simulink model "quaternion_attitude_control_nominal"  (R2024b)
settings: Solver=ode45  StartTime=0.0  StopTime=1500  MaxStep=0.2
values from neighbouring files (symbols this model uses):
  Cross_section_area = 0.01    [init_conditions.m]
  d = 0.8    [init_conditions.m]
  finalAttitude = [-1/sqrt(2); 0; 0; -1/sqrt(2)]    [init_conditions.m]
  J = calculateInertiaTensor(mass, sideLength)    [init_conditions.m]
  k = 0.32    [init_conditions.m]
  mass = 1.33    [init_conditions.m]
undefined symbols (not defined in the file or in its folder): compute_drag
libraries: aerolibutil x2, aerolibgravity2 x1
settings Model: VariantFading=off  LastModifiedBy=shavykashyap
settings SolverCC: ZeroCrossAlgorithm=Adaptive
settings DataIOCC: Refine=2
settings DebuggingCC: MaskedZcDiagnostic=none  IgnoredZcDiagnostic=none

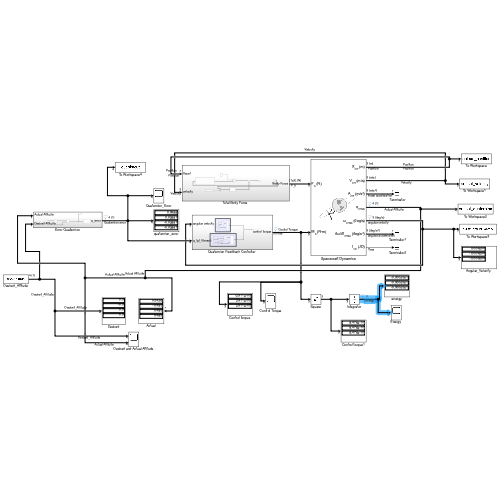
[thumbnail: Simulink's stored preview of the top-level diagram]
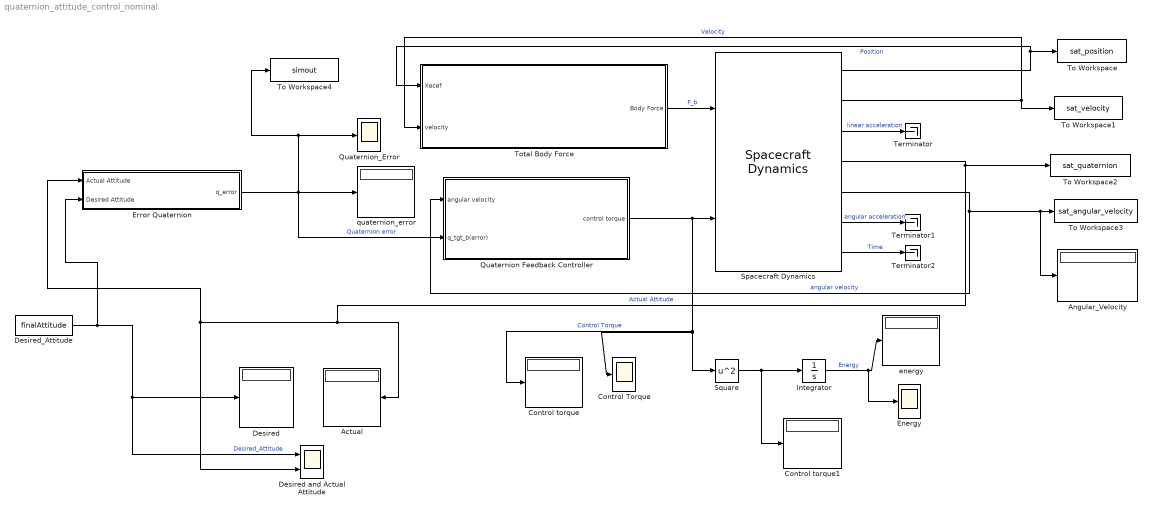
== system quaternion_attitude_control_nominal ==
  Actual : Display
  "Angular_Velocity " : Display
  Control Torque : Scope
  Control torque : Display
  Control torque1 : Display
  Desired : Display
  Desired and Actual Attitude : Scope  NumInputPorts=2
  Desired_Attitude : Constant  Value=finalAttitude
  Energy : Scope
  Error Quaternion : Subsystem
  Integrator : Integrator
  "Quaternion Feedback Controller " : Subsystem
  Quaternion_Error : Scope
  Spacecraft Dynamics : SpacecraftDynamics  outputAccel=on  mass=mass  inertia=J  stateFormatNum=ICRF state vector  inertialPosition=initialPosition  inertialVelocity=initialVelocity  attitude=initialAttitude  attitudeRate=initialAngularVelocity  outputAngAccel=on  gravityModel=Oblate ellipsoid (J2)  useDrag=on  useSRP=on
  Square : Math  Operator=square
  Terminator : Terminator
  Terminator1 : Terminator
  Terminator2 : Terminator
  To Workspace : ToWorkspace  VariableName=sat_position  SaveFormat=Timeseries  SampleTime=-1
  To Workspace1 : ToWorkspace  VariableName=sat_velocity  SaveFormat=Timeseries  SampleTime=-1
  To Workspace2 : ToWorkspace  VariableName=sat_quaternion  SaveFormat=Timeseries  SampleTime=-1
  To Workspace3 : ToWorkspace  VariableName=sat_angular_velocity  SaveFormat=Timeseries  SampleTime=-1
  To Workspace4 : ToWorkspace  VariableName=simout  SaveFormat=Timeseries  SampleTime=-1
  "Total Body Force " : Subsystem
  energy : Display
  quaternion_error : Display
  wires:
  Spacecraft Dynamics/1 -> "Total Body Force "/1(Xecef), To Workspace/1  "Position"
  Spacecraft Dynamics/2 -> To Workspace1/1, "Total Body Force "/2(velocity)  "Velocity"
  Spacecraft Dynamics/4 -> Desired and Actual Attitude/2, Error Quaternion/1(Actual Attitude), Actual/1, To Workspace2/1  "Actual Attitude"
  Spacecraft Dynamics/5 -> "Quaternion Feedback Controller "/1(angular velocity), "Angular_Velocity "/1, To Workspace3/1  "angular velocity"
  "Quaternion Feedback Controller "/1(control torque) -> Square/1, Control Torque/1, Control torque/1, Spacecraft Dynamics/2  "Control Torque"
  Desired_Attitude/1 -> Error Quaternion/2(Desired Attitude), Desired and Actual Attitude/1, Desired/1  "Desired_Attitude"
  Spacecraft Dynamics/6 -> Terminator1/1  "angular acceleration"
  Spacecraft Dynamics/7 -> Terminator2/1  "Time"
  Spacecraft Dynamics/3 -> Terminator/1  "linear acceleration"
  "Total Body Force "/1(Body Force) -> Spacecraft Dynamics/1  "F_b"
  Error Quaternion/1(q_error) -> "Quaternion Feedback Controller "/2(q_tgt_b(error)), To Workspace4/1, Quaternion_Error/1, quaternion_error/1  "Quaternion error"
  Square/1 -> Control torque1/1, Integrator/1
  Integrator/1 -> Energy/1, energy/1  "Energy"

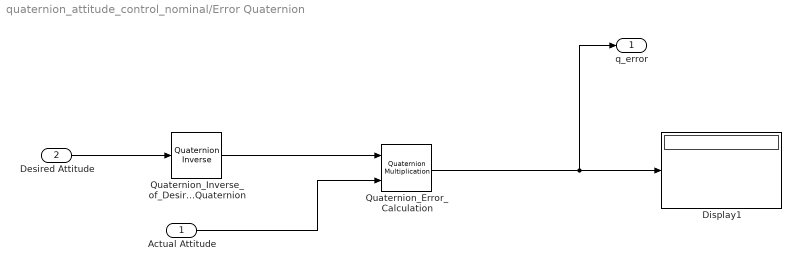
== system quaternion_attitude_control_nominal/Error Quaternion ==
  Actual Attitude : Inport
  Desired Attitude : Inport  Port=2
  Display1 : Display
  Quaternion_Error_Calculation : aerolibutil/Quaternion Multiplication
  Quaternion_Inverse_of_Desired_Quaternion : aerolibutil/Quaternion Inverse
  q_error : Outport
  wires:
  Actual Attitude/1 -> Quaternion_Error_Calculation/2
  Quaternion_Inverse_of_Desired_Quaternion/1 -> Quaternion_Error_Calculation/1
  Desired Attitude/1 -> Quaternion_Inverse_of_Desired_Quaternion/1
  Quaternion_Error_Calculation/1 -> q_error/1, Display1/1

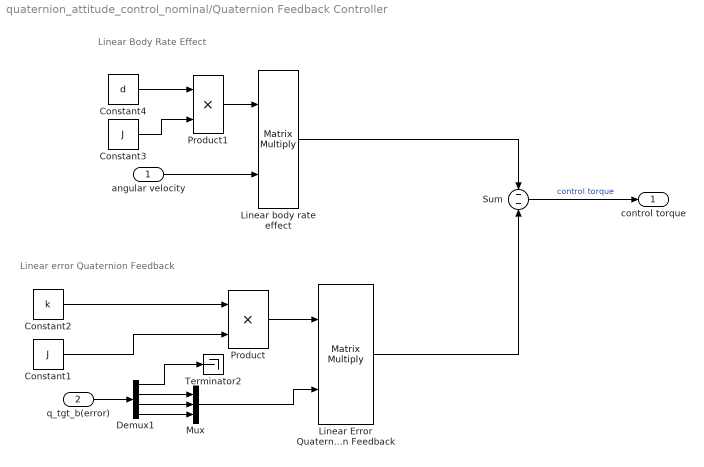
== system quaternion_attitude_control_nominal/Quaternion Feedback Controller  ==
  note: Linear error Quaternion Feedback
  note: Linear Body Rate Effect
  angular velocity : Inport
  q_tgt_b(error) : Inport  Port=2
  Constant1 : Constant  Value=J
  Constant2 : Constant  Value=k
  Constant3 : Constant  Value=J
  Constant4 : Constant  Value=d
  Demux1 : Demux
  Linear Error Quaternion Feedback : Product  Multiplication=Matrix(*)
  Linear body rate effect : Product  Multiplication=Matrix(*)
  Mux : Mux  Inputs=3
  Product : Product
  Product1 : Product
  Sum : Sum  Inputs=--
  Terminator2 : Terminator
  control torque : Outport
  wires:
  Linear body rate effect/1 -> Sum/1
  Mux/1 -> Linear Error Quaternion Feedback/2
  angular velocity/1 -> Linear body rate effect/2
  Demux1/1 -> Terminator2/1
  Constant1/1 -> Product/2
  Linear Error Quaternion Feedback/1 -> Sum/2
  Demux1/4 -> Mux/3
  Constant2/1 -> Product/1
  Demux1/2 -> Mux/1
  Demux1/3 -> Mux/2
  Constant3/1 -> Product1/2
  q_tgt_b(error)/1 -> Demux1/1
  Sum/1 -> control torque/1  "control torque"
  Constant4/1 -> Product1/1
  Product/1 -> Linear Error Quaternion Feedback/1
  Product1/1 -> Linear body rate effect/1

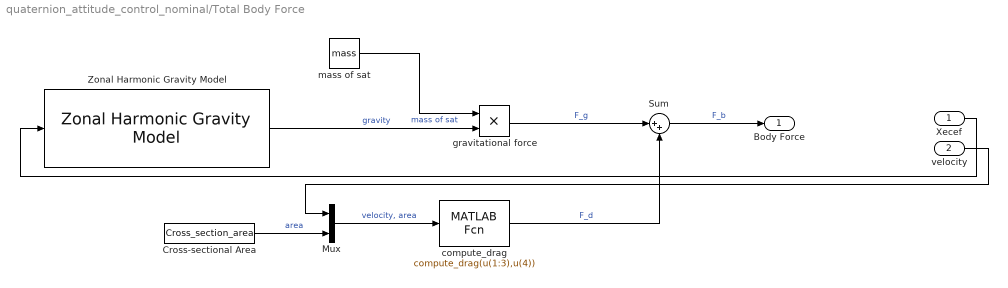
== system quaternion_attitude_control_nominal/Total Body Force  ==
  Xecef : Inport
  velocity : Inport  Port=2
  Cross-sectional Area : Constant  Value=Cross_section_area
  Mux : Mux  Inputs=2
  Sum : Sum  Inputs=|++
  Zonal Harmonic Gravity Model : aerolibgravity2/Zonal Harmonic Gravity Model  units=Metric (MKS)  degree=4  action=Warning  ptype=Earth  R=6378136.3  GM=398600441500000  jvalue=[1.0826269e-03 -2.5323000e-06 -1.6204000e-06]
  compute_drag : MATLABFcn  MATLABFcn=compute_drag(u(1:3),u(4))
  gravitational force : Product
  mass of sat : Constant  Value=mass
  Body Force : Outport
  wires:
  mass of sat/1 -> gravitational force/1  "mass of sat"
  compute_drag/1 -> Sum/2  "F_d"
  Mux/1 -> compute_drag/1  "velocity, area"
  Cross-sectional Area/1 -> Mux/2  "area"
  gravitational force/1 -> Sum/1  "F_g"
  Zonal Harmonic Gravity Model/1 -> gravitational force/2  "gravity"
  Xecef/1 -> Zonal Harmonic Gravity Model/1
  Sum/1 -> Body Force/1  "F_b"
  velocity/1 -> Mux/1
